simulink model "simulacion_tanqueAgua_completo"  (R2026b)
settings: Solver=VariableStepAuto  StopTime=50
undefined symbols (not defined in the file): A, h0, Hmax, K, tStep
settings Model: LastModifiedBy=Yenderson Josué

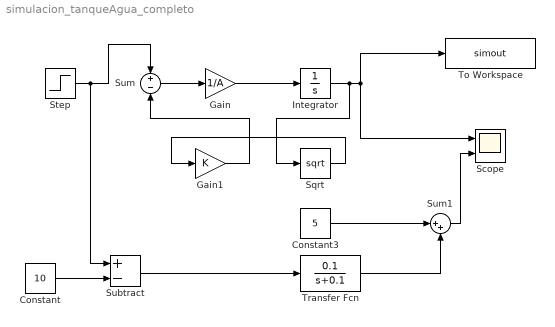
== system simulacion_tanqueAgua_completo ==
  Constant : Constant  Value=10
  Constant3 : Constant  Value=5
  Gain : Gain  Gain=1/A
  Gain1 : Gain  Gain=K
  Integrator : Integrator  InitialCondition=h0  LimitOutput=on  UpperSaturationLimit=Hmax  LowerSaturationLimit=0
  Scope : Scope  NumInputPorts=2
      settings: ActiveDisplayYMinimum=-0.89689148505529348  ActiveDisplayYMaximum=8.0720233654976425
  Sqrt : Sqrt
  Step : Step  Time=tStep  InitialValue=Qi0  FinalValue=Qi1  SampleTime=0
  Subtract : Sum  Inputs=+-
  Sum : Sum  Inputs=+-
  Sum1 : Sum  Inputs=|++
  To Workspace : ToWorkspace  VariableName=simout  SaveFormat=Timeseries  SampleTime=-1
  Transfer Fcn : TransferFcn  Numerator=[0.1]  Denominator=[1 0.1]
  wires:
  Step/1 -> Subtract/1, Sum/1
  Sum/1 -> Gain/1
  Gain/1 -> Integrator/1
  Integrator/1 -> Sqrt/1, To Workspace/1, Scope/1
  Sqrt/1 -> Gain1/1
  Gain1/1 -> Sum/2
  Constant/1 -> Subtract/2
  Subtract/1 -> Transfer Fcn/1
  Constant3/1 -> Sum1/1
  Transfer Fcn/1 -> Sum1/2
  Sum1/1 -> Scope/2
